simulink model "CubeSat_Simulator"  (R2019a)
settings: Solver=ode4  StartTime=0.0  StopTime=54000  FixedStep=0.1  RelTol=1e-5
model workspace: external: MATLAB File C:\Users\Heyang Zhang\OneDrive\02_Education\01_Undergraduate\02_Capstone\Killick-1 CubeSat\05_Technical\01_Simulation\01_Killick1\Simscape\Killick1_simScape_DataFile.m (data not in the file)
values from neighbouring files (symbols this model uses):
  a_desired = 0.35    [CubeSat_Parameter.m]
  D_distri = G_s.'* inv(G_s * G_s.')    [CubeSat_Parameter.m]
  G_s = [-cos(a_inc)*sin(b_rot)  -cos(a_inc)*cos(b_rot)   cos(a_inc)*sin(b_rot)  cos(a_inc)*cos(b_rot) ... (first row only)    [CubeSat_Parameter.m]
  I_rw = I_s - sum_rw    [CubeSat_Parameter.m]
  I_w = [3500E-9  3500E-9  3500E-9  3500E-9 ... (first row only)    [CubeSat_Parameter.m]
  Kc = [eye(3).*[2.5;2.5;2.5]  eye(3).*[5;5;5]]    [CubeSat_Parameter.m]
  Ki = [eye(3).*[1.2 1.2 1.2]  eye(3).*[3;3;3]]    [CubeSat_Parameter.m]
  Kw_d = 0.4    [CubeSat_Parameter.m]
  Kw_i = 0.1    [CubeSat_Parameter.m]
  Kw_p = 0.4    [CubeSat_Parameter.m]
  OMEGA_0 = [0;0;0]    [CubeSat_Parameter.m]
  quat_0 = eul2quat(eulr_0).'    [CubeSat_Parameter.m]
  SatMass = 3.5    [CubeSat_Parameter.m]
  tau_sat_mt = 1e-3    (= 0.001)    [CubeSat_Parameter.m]
  tau_sat_rw = 5e-3    (= 0.005)    [CubeSat_Parameter.m]
  w_desired = 0.35    [CubeSat_Parameter.m]
  w_rw_ref = [0;0;-0;-0]    [CubeSat_Parameter.m]
undefined symbols (not defined in the file or in its folder): Earth, IAU, km, Kp, Kv, s, WGS84
libraries: sharedutil x19, aerolibutil x18, dspmathops x18, sharedtransform x13, simulink_extras x8, aerolibtransform2 x5, simulink x5, asbCubeSatBlockLib x5, aerolibconvert2 x3, dsparch4 x3, ADCS_lib x2, aerolibcelestial x2
(part 3 of 3)

== system CubeSat_Simulator/GNC Computer/Guidance/Trajectory Planning/Spatial Rotation to Quaternion ==
  PRA : Inport
  PRV : Inport  Port=2
  Gain1 : Gain  Gain=0.5
  Mux : Mux  Inputs=2
  Product : Product
  Trigonometric Function2 : Trigonometry  Operator=cos
  Trigonometric Function3 : Trigonometry  OutputSignalType=real
  q : Outport
  wires:
  PRA/1 -> Gain1/1
  Gain1/1 -> Trigonometric Function3/1, Trigonometric Function2/1
  Trigonometric Function2/1 -> Mux/1
  Trigonometric Function3/1 -> Product/1
  PRV/1 -> Product/2
  Product/1 -> Mux/2
  Mux/1 -> q/1

== system CubeSat_Simulator/GNC Computer/Guidance/Trapzodial Velocity Profile/key time stamp ==
  p_input : Inport
  v_input : Inport  Port=2
  a_input : Inport  Port=3
  Add : Sum  Inputs=+-
  Add1 : Sum  Inputs=|+-
  Divide : Product  Inputs=*/
  Divide1 : Product  Inputs=*/
  Divide2 : Product  Inputs=*/
  Math Function : Math  Operator=square  SaturateOnIntegerOverflow=on
  Product : Product
  Sqrt : Sqrt  SaturateOnIntegerOverflow=on
  check if w_desired>w_max : Switch  Criteria=u2 > Threshold
  p : Outport
  v : Outport  Port=2
  a : Outport  Port=3
  t_acc : Outport  Port=4
  t_cst : Outport  Port=5
  t_dcl : Outport  Port=6
  wires:
  Add/1 -> check if w_desired>w_max/2
  Add1/1 -> Divide1/1
  Sqrt/1 -> check if w_desired>w_max/3, Add/1  "w_max"
  v_input/1 -> check if w_desired>w_max/1, Add/2
  Math Function/1 -> Divide/1
  check if w_desired>w_max/1 -> v/1, Divide2/1, Math Function/1, Divide1/2  "w"
  p_input/1 -> p/1, Add1/1, Product/1
  a_input/1 -> a/1, Divide2/2, Product/2, Divide/2
  Divide1/1 -> t_cst/1
  Divide/1 -> Add1/2
  Product/1 -> Sqrt/1
  Divide2/1 -> t_dcl/1, t_acc/1

== system CubeSat_Simulator/GNC Computer/Control/LQI_Full State_Verified/Vector Out Unwinding1/Short Rotation ==
  q : Inport
  Gain1 : Gain  Gain=-1
  Sign1 : Signum
  extract scalar part : Selector  InputPortWidth=4  IndexOptions=Index vector (dialog)  Indices=[1]  OutputSizes=1
  sgn : Outport
  wires:
  Gain1/1 -> sgn/1
  Sign1/1 -> Gain1/1
  extract scalar part/1 -> Sign1/1
  q/1 -> extract scalar part/1

== matlab function CubeSat_Simulator/GNC Computer/Control/PIV Full EoM/Cross Product ==
  data: u input; u_tilde output
function u_tilde = tilde(u)
u_tilde = [0 -u(3) u(2);
           u(3) 0 -u(1);
           -u(2) u(1) 0];

== matlab function CubeSat_Simulator/Visualize/MATLAB Function ==
  data: u input; y output
function y = norm(u)

y = norm(u);

== matlab function CubeSat_Simulator/GNC Computer/Guidance/Trapzodial Velocity Profile/MATLAB Function ==
  data: p input; v input; a input; T1 input; p_traj output; T2 input; T3 input; v_traj output; a_traj output
function [p_traj,v_traj,a_traj]= fcn(p,v,a,T1,T2,T3)

% row time vctr, initial time:step size:final time
Ts = 0.001;
tau1 = 0:Ts:T1;
tau2 = 0:Ts:T2;
tau3 = 0:Ts:T3;

% initialize array for three stages
pos1 = zeros(1,length(tau1));
vel1 = zeros(1,length(tau1));
acc1 = zeros(1,length(tau1));

pos2 = zeros(1,length(tau2));
vel2 = zeros(1,length(tau2));
acc2 = zeros(1,length(tau2));

pos3 = zeros(1,length(tau3));
vel3 = zeros(1,length(tau3));
acc3 = zeros(1,length(tau3));

% calculate pos,vel,acc for three stages
for i = 1:length(tau1) % accelerating
    pos1(i) = v*tau1(i)*tau1(i)/2/T1;
    vel1(i) = v*tau1(i)/T1;
    acc1(i) = a;
end
for i = 1:length(tau2) % coasting
    pos2(i) = v*tau2(i)+v*T1/2;
    vel2(i) = v;
    acc2(i) = 0;
end
for i = 1:length(tau3) % coasting
    pos3(i) = -v*tau3(i)*tau3(i)/2/T3+v*tau3(i)+p-v*T3/2;
    vel3(i) = -v*tau3(i)/T3+v;
    acc3(i) = -a;
end

p_traj = [pos1 pos2 pos3];
v_traj = [vel1 vel2 vel3];
a_traj = [acc1 acc2 acc3];

== matlab function CubeSat_Simulator/GNC Computer/Guidance/Trapzodial Velocity Profile/MATLAB Function1 ==
  data: v input; a input; T1 input; y output
function y= fcn(v,a,T1)

dt = 0.001; % time step
step1 = round(T1/0.001); % how many time steps in one given number of time period

for i = 1:step1 % accelerating
    pos1(i) = v*tau1(i)*tau1(i)/2/T1;
    vel1(i) = v*tau1(i)/T1;
    acc1(i) = a;
end

% initialize array for three stages
% pos1 = zeros(1,length(tau1));
% vel1 = zeros(1,length(tau1));
% acc1 = zeros(1,length(tau1));
% 
% pos2 = zeros(1,length(tau2));
% vel2 = zeros(1,length(tau2));
% acc2 = zeros(1,length(tau2));
% 
% pos3 = zeros(1,length(tau3));
% vel3 = zeros(1,length(tau3));
% acc3 = zeros(1,length(tau3));
% 
% % calculate pos,vel,acc for three stages
% for i = 1:length(tau1) % accelerating
%     pos1(i) = v*tau1(i)*tau1(i)/2/T1;
%     vel1(i) = v*tau1(i)/T1;
%     acc1(i) = a;
% end
% for i = 1:length(tau2) % coasting
%     pos2(i) = v*tau2(i)+v*T1/2;
%     vel2(i) = v;
%     acc2(i) = 0;
% end
% for i = 1:length(tau3) % coasting
%     pos3(i) = -v*tau3(i)*tau3(i)/2/T3+v*tau3(i)+p-v*T3/2;
%     vel3(i) = -v*tau3(i)/T3+v;
%     acc3(i) = -a;
% end
% 
% p_traj = [pos1 pos2 pos3];
% v_traj = [vel1 vel2 vel3];
% a_traj = [acc1 acc2 acc3];

== matlab function CubeSat_Simulator/Environment/External Force and Torque/MATLAB Function ==
  data: rho_atm input; w_earth_eci input; x_eci input; f_aero_body output; v_eci input; q_eci2body input; t_aero_body output; faceArea parameter; dragCoeff parameter; cpLocation parameter; faceNormal parameter
function [f_aero_body,t_aero_body]= AeroPtrb(rho_atm,w_earth_eci,x_eci,v_eci,q_eci2body,faceArea,dragCoeff,cpLocation,faceNormal)
faceNumber = size(faceNormal,2);
incl = zeros(1,faceNumber);
f_aero = zeros(3,faceNumber);
t_aero = zeros(3,faceNumber);
v_rel_eci = v_eci + cross(w_earth_eci,x_eci);
v_rel_body = (quat2rotm(q_eci2body'))'*v_rel_eci;
for i = 1:faceNumber
    incl(:,i) = (dot(faceNormal(:,i),v_rel_body))/(norm(v_eci));
    f_aero(:,i) = -0.5*rho_atm*dragCoeff(i)*norm(v_eci)...
                  *v_rel_body*faceArea(i)*max(incl(:,i),0);
    t_aero(:,i) = cross(cpLocation(:,i),f_aero(:,i));
end
f_aero_body = sum(f_aero,2);
t_aero_body = sum(t_aero,2);

== matlab function CubeSat_Simulator/Environment/External Force and Torque/Exp Decay Air Density/MATLAB Function3 ==
  data: h input; h_0 input; rho output; rho_0 input; H input
function rho = Density(h,h_0,rho_0,H)

rho = rho_0*exp(-((h-h_0)/(H)))
